simulink model "SpwmTHIpwm"  (R2018a)
settings: Solver=FixedStepDiscrete  StartTime=0.0  StopTime=1  FixedStep=1e-6  RelTol=1e-3
values from neighbouring files (symbols this model uses):
  A_3 = 1/6    (= 0.166666666667)    [SpwmTpwm.m]
  A_c = 1    [SpwmTpwm.m]
  f_c = 5e4    (= 50000)    [PWM.m]    (also in SpaceVector.m = 50; SpwmTpwm.m = 50)
  f_s = 10000    [SpaceVector.m]    (also in SpaceVectorOnlyCode.m = 1000; SpwmTpwm.m)
  V_dc = 100    [SpaceVector.m]    (also in SpaceVectorOnlyCode.m = 500; SpwmTpwm.m)
libraries: peGeneralControl x3, simulink x1
settings Model: Creator=enes_  LastModifiedBy=enes_

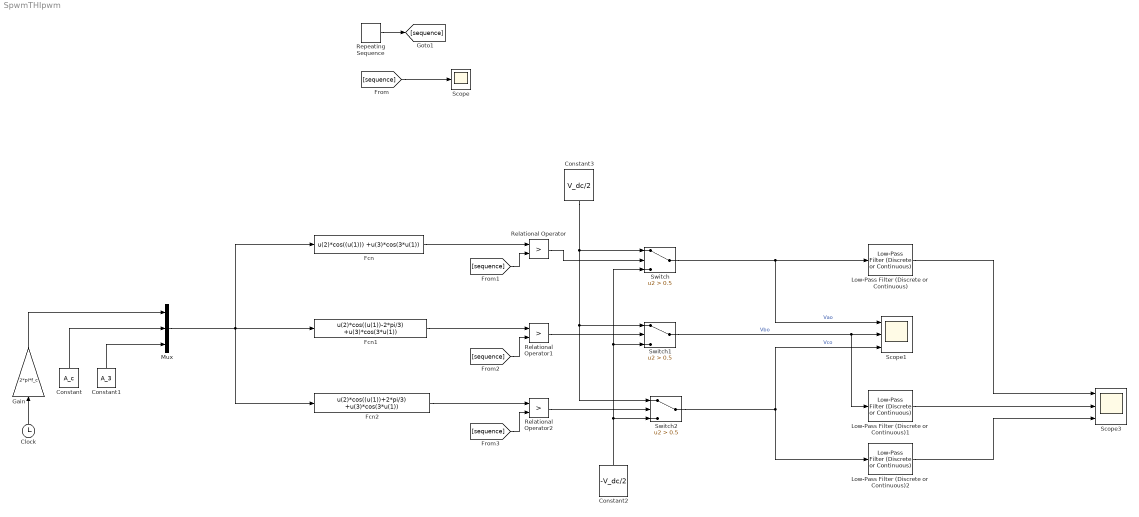
== system SpwmTHIpwm ==
  Clock : Clock
  Constant : Constant  Value=A_c
  Constant1 : Constant  Value=A_3
  Constant2 : Constant  Value=-V_dc/2
  Constant3 : Constant  Value=V_dc/2
  Fcn : Fcn  Expr=u(2)*cos((u(1))) +u(3)*cos(3*u(1))
  Fcn1 : Fcn  Expr=u(2)*cos((u(1))-2*pi/3) +u(3)*cos(3*u(1))
  Fcn2 : Fcn  Expr=u(2)*cos((u(1))+2*pi/3) +u(3)*cos(3*u(1))
  Gain : Gain  Gain=2*pi*f_c
  Low-Pass Filter (Discrete or Continuous) : peGeneralControl/Low-Pass Filter (Discrete or Continuous)  K=8  T=20e-3  B=inf  A=-inf  Ts=-1
  Low-Pass Filter (Discrete or Continuous)1 : peGeneralControl/Low-Pass Filter (Discrete or Continuous)  K=8  T=20e-3  B=inf  A=-inf  Ts=-1
  Low-Pass Filter (Discrete or Continuous)2 : peGeneralControl/Low-Pass Filter (Discrete or Continuous)  K=8  T=20e-3  B=inf  A=-inf  Ts=-1
  Mux : Mux  Inputs=3
  Relational Operator : RelationalOperator  Operator=>  OutDataTypeStr=boolean  RndMeth=Simplest
  Relational Operator1 : RelationalOperator  Operator=>  OutDataTypeStr=boolean  RndMeth=Simplest
  Relational Operator2 : RelationalOperator  Operator=>  OutDataTypeStr=boolean  RndMeth=Simplest
  Repeating Sequence : simulink/Sources/Repeating Sequence  rep_seq_t=[0 1 2 3 4] /f_s  rep_seq_y=[-1 0 1 0 -1]
  Scope : Scope
  Scope1 : Scope  NumInputPorts=3
  Scope3 : Scope  NumInputPorts=3
  Switch : Switch  Criteria=u2 > Threshold  Threshold=0.5
  Switch1 : Switch  Criteria=u2 > Threshold  Threshold=0.5
  Switch2 : Switch  Criteria=u2 > Threshold  Threshold=0.5
  wires:
  Clock/1 -> Gain/1
  Constant/1 -> Mux/2
  Gain/1 -> Mux/1
  Constant1/1 -> Mux/3
  Mux/1 -> Fcn1/1, Fcn2/1, Fcn/1
  Repeating Sequence/1 -> [sequence]
  [sequence] -> Scope/1
  Fcn/1 -> Relational Operator/1
  Fcn1/1 -> Relational Operator1/1
  Fcn2/1 -> Relational Operator2/1
  [sequence] -> Relational Operator/2
  [sequence] -> Relational Operator1/2
  [sequence] -> Relational Operator2/2
  Relational Operator/1 -> Switch/2
  Relational Operator1/1 -> Switch1/2
  Relational Operator2/1 -> Switch2/2
  Constant3/1 -> Switch/1, Switch1/1, Switch2/1
  Constant2/1 -> Switch2/3, Switch1/3, Switch/3
  Switch1/1 -> Low-Pass Filter (Discrete or Continuous)1/1, Scope1/2  "Vbo"
  Switch/1 -> Low-Pass Filter (Discrete or Continuous)/1, Scope1/1  "Vao"
  Switch2/1 -> Low-Pass Filter (Discrete or Continuous)2/1, Scope1/3  "Vco"
  Low-Pass Filter (Discrete or Continuous)/1 -> Scope3/1
  Low-Pass Filter (Discrete or Continuous)1/1 -> Scope3/2
  Low-Pass Filter (Discrete or Continuous)2/1 -> Scope3/3
